simulink model "tester"  (R2022b)
settings: Solver=VariableStepAuto  StartTime=0.0  StopTime=45  RelTol=1e-3
values from neighbouring files (symbols this model uses):
  ACCtime = 0    [dane.m]    (also in szybkiwykres.m; wykresownikfinalny.m)
  E4time = 700    [dane.m]
settings Model: Creator=48519  LastModifiedBy=48519
settings ModelReferenceCC: EnableRefExpFcnMdlSchedulingChecks=on

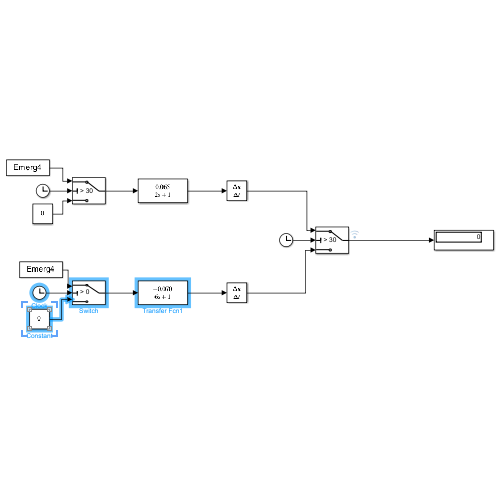
[thumbnail: Simulink's stored preview of the top-level diagram]
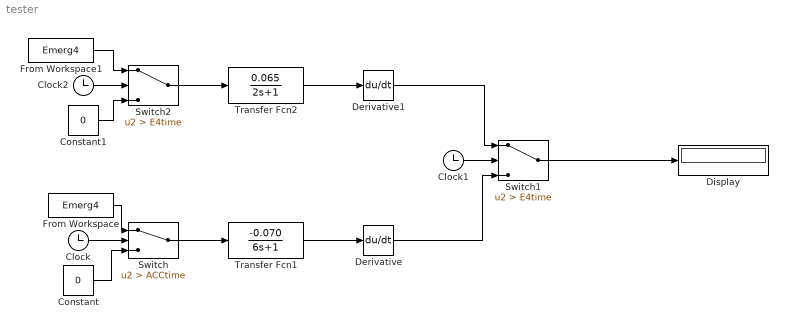
== system tester ==
  Clock : Clock
  Clock1 : Clock
  Clock2 : Clock
  Constant : Constant  Value=0
  Constant1 : Constant  Value=0
  Derivative : Derivative
  Derivative1 : Derivative
  Display : Display
  From Workspace : FromWorkspace  VariableName=Emerg4
  From Workspace1 : FromWorkspace  VariableName=Emerg4
  Switch : Switch  Criteria=u2 > Threshold  Threshold=ACCtime  SaturateOnIntegerOverflow=off  InputSameDT=off
  Switch1 : Switch  Criteria=u2 > Threshold  Threshold=E4time  SaturateOnIntegerOverflow=off  InputSameDT=off
  Switch2 : Switch  Criteria=u2 > Threshold  Threshold=E4time  SaturateOnIntegerOverflow=off  InputSameDT=off
  Transfer Fcn1 : TransferFcn  Numerator=[-0.070]  Denominator="[6  1]"
  Transfer Fcn2 : TransferFcn  Numerator=[0.065]  Denominator="[2  1]"
  wires:
  Switch2/1 -> Transfer Fcn2/1
  Clock/1 -> Switch/2
  Clock2/1 -> Switch2/2
  Derivative/1 -> Switch1/3
  Clock1/1 -> Switch1/2
  Constant/1 -> Switch/3
  Switch/1 -> Transfer Fcn1/1
  From Workspace1/1 -> Switch2/1
  Constant1/1 -> Switch2/3
  From Workspace/1 -> Switch/1
  Transfer Fcn2/1 -> Derivative1/1
  Transfer Fcn1/1 -> Derivative/1
  Derivative1/1 -> Switch1/1
  Switch1/1 -> Display/1
